simulink model "Work3"  (R2015b)
settings: Solver=FixedStepAuto  SolverMode=SingleTasking  StartTime=0.0  StopTime=20  FixedStep=0.01  RelTol=1e-3
values from neighbouring files (symbols this model uses):
  diff = 4    [diff.mat]
  diff2 = 240    [diff2.mat]
  Integ = 1.89    [Integ.mat]
  Integ2 = 1.6    [Integ2.mat]
  P = 8    [P.mat]
  P2 = 360    [P2.mat]
undefined symbols (not defined in the file or in its folder): ss1, ss2
settings Model: ExtModeTrigDuration=2  Creator=Druzhinin_Vasily  LastModifiedBy=Druzhinin_Vasily
settings OptimizationCC: DefaultParameterBehavior=Inlined  UseFloatMulNetSlope=on  InlineInvariantSignals=on  PassReuseOutputArgsAs=Individual arguments  ZeroExternalMemoryAtStartup=off  ZeroInternalMemoryAtStartup=off  NoFixptDivByZeroProtection=on  EfficientFloat2IntCast=on  OptimizeModelRefInitCode=on  LifeSpan=1  MaxStackSize=64
settings RTWCC: SystemTargetFile=ert.tlc  TemplateMakefile=ert_default_tmf  Description=Embedded Coder  GenerateReport=on  Toolchain=Arduino AVR v1.6.1  BuildConfiguration=Faster Runs  IncludeHyperlinkInReport=on  LaunchReport=on  GenerateTraceInfo=on  GenerateTraceReport=on  GenerateTraceReportSl=on  GenerateTraceReportSf=on  GenerateTraceReportEml=on  GenerateCodeMetricsReport=on
settings CodeAppCC: ForceParamTrailComments=on  IgnoreCustomStorageClasses=off  SimulinkDataObjDesc=on  CustomSymbolStrGlobalVar=rt$N$M  CustomSymbolStrType=$N$M  CustomSymbolStrFcn=$N$M$F  CustomSymbolStrMacro=$N$M  InsertBlockDesc=on
settings ERTTargetCC: IncludeMdlTerminateFcn=off  CombineSignalStateStructs=on  SupportContinuousTime=on  SupportVariableSizeSignals=on  InlinedParameterPlacement=NonHierarchical  ERTCustomFileTemplate=example_file_process.tlc  ERTFilePackagingFormat=CompactWithDataFile

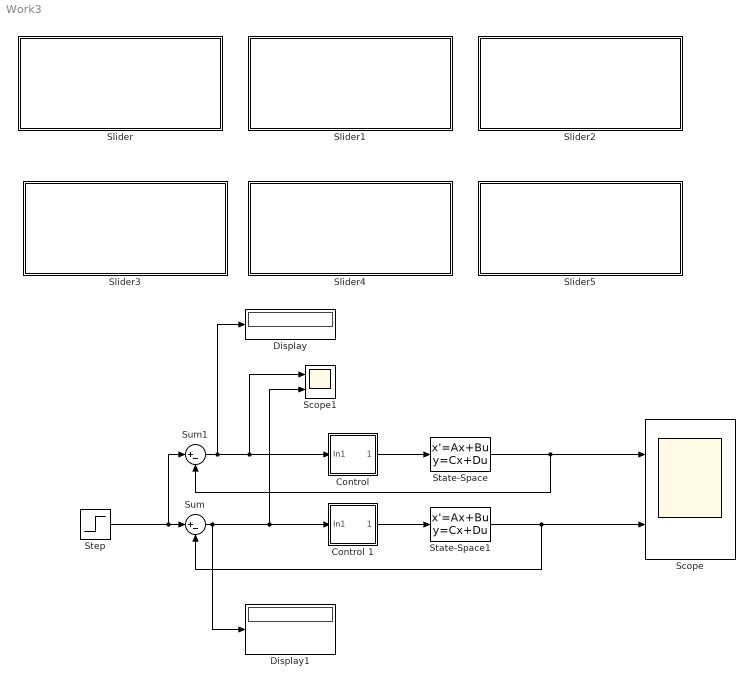
== system Work3 ==
  "Control " : Subsystem
  Control 1 : Subsystem
  Display : Display
  Display1 : Display
  Scope : Scope  NumInputPorts=2
  Scope1 : Scope  NumInputPorts=2
  Slider : Subsystem  DialogController=hmiCreateDDGDialog  IsWebBlock=on  mask(MWDashboardBlock){webBlockId=fcde2a52-5679-498e-b0b0-f5f8bdaff23e, webBlockType=slider, ShowInLibBrowser=on, ShowInitialText=on, HMISrcModelName=Work3}
      mask prompts: webBlockId "WebBlock Id"; webBlockType "WebBlock Type"; HMISrcModelName "Source Model"
      mask Help: helpview([docroot '/mapfiles/simulink.map'], 'hmi_slider')
      mask Display:
      | if strcmp(get_param(bdroot(gcb),'BlockDiagramType'), 'library')
      |     image([(matlabroot) '/toolbox/simulink/hmi/icons/Slider.png']);
      | end
  Slider1 : Subsystem  DialogController=hmiCreateDDGDialog  IsWebBlock=on  mask(MWDashboardBlock){webBlockId=34f26c4b-778d-474b-b420-5e3debdaa527, webBlockType=slider, ShowInLibBrowser=on, ShowInitialText=on, HMISrcModelName=Work3}
      mask prompts: webBlockId "WebBlock Id"; webBlockType "WebBlock Type"; HMISrcModelName "Source Model"
      mask Help: helpview([docroot '/mapfiles/simulink.map'], 'hmi_slider')
      mask Display:
      | if strcmp(get_param(bdroot(gcb),'BlockDiagramType'), 'library')
      |     image([(matlabroot) '/toolbox/simulink/hmi/icons/Slider.png']);
      | end
  Slider2 : Subsystem  DialogController=hmiCreateDDGDialog  IsWebBlock=on  mask(MWDashboardBlock){webBlockId=5f60686c-b0fe-4f18-a9e2-fcd4e663f137, webBlockType=slider, ShowInLibBrowser=on, ShowInitialText=on, HMISrcModelName=Work3}
      mask prompts: webBlockId "WebBlock Id"; webBlockType "WebBlock Type"; HMISrcModelName "Source Model"
      mask Help: helpview([docroot '/mapfiles/simulink.map'], 'hmi_slider')
      mask Display:
      | if strcmp(get_param(bdroot(gcb),'BlockDiagramType'), 'library')
      |     image([(matlabroot) '/toolbox/simulink/hmi/icons/Slider.png']);
      | end
  Slider3 : Subsystem  DialogController=hmiCreateDDGDialog  IsWebBlock=on  mask(MWDashboardBlock){webBlockId=a2bf55c6-834c-4e95-99ad-44c455448221, webBlockType=slider, ShowInLibBrowser=on, ShowInitialText=on, HMISrcModelName=Work3}
      mask prompts: webBlockId "WebBlock Id"; webBlockType "WebBlock Type"; HMISrcModelName "Source Model"
      mask Help: helpview([docroot '/mapfiles/simulink.map'], 'hmi_slider')
      mask Display:
      | if strcmp(get_param(bdroot(gcb),'BlockDiagramType'), 'library')
      |     image([(matlabroot) '/toolbox/simulink/hmi/icons/Slider.png']);
      | end
  Slider4 : Subsystem  DialogController=hmiCreateDDGDialog  IsWebBlock=on  mask(MWDashboardBlock){webBlockId=93ab61cf-ceae-4acd-b5ad-db12f044e680, webBlockType=slider, ShowInLibBrowser=on, ShowInitialText=on, HMISrcModelName=Work3}
      mask prompts: webBlockId "WebBlock Id"; webBlockType "WebBlock Type"; HMISrcModelName "Source Model"
      mask Help: helpview([docroot '/mapfiles/simulink.map'], 'hmi_slider')
      mask Display:
      | if strcmp(get_param(bdroot(gcb),'BlockDiagramType'), 'library')
      |     image([(matlabroot) '/toolbox/simulink/hmi/icons/Slider.png']);
      | end
  Slider5 : Subsystem  DialogController=hmiCreateDDGDialog  IsWebBlock=on  mask(MWDashboardBlock){webBlockId=0c8f17bd-0089-4b6b-8033-3296dc0310bd, webBlockType=slider, ShowInLibBrowser=on, ShowInitialText=on, HMISrcModelName=Work3}
      mask prompts: webBlockId "WebBlock Id"; webBlockType "WebBlock Type"; HMISrcModelName "Source Model"
      mask Help: helpview([docroot '/mapfiles/simulink.map'], 'hmi_slider')
      mask Display:
      | if strcmp(get_param(bdroot(gcb),'BlockDiagramType'), 'library')
      |     image([(matlabroot) '/toolbox/simulink/hmi/icons/Slider.png']);
      | end
  State-Space : StateSpace  A=ss1.A  B=ss1.B  C=ss1.C  D=ss1.D  X0=0
  State-Space1 : StateSpace  A=ss2.A  B=ss2.B  C=ss2.C  D=ss2.D  X0=0
  Step : Step  SampleTime=0
  Sum : Sum  Inputs=|+-
  Sum1 : Sum  Inputs=|+-
  wires:
  State-Space/1 -> Sum1/2, Scope/1
  Step/1 -> Sum/1, Sum1/1
  State-Space1/1 -> Sum/2, Scope/2
  Sum/1 -> Display1/1, Control 1/1(In1), Scope1/2
  Sum1/1 -> Display/1, "Control "/1(In1), Scope1/1
  Control 1/1(Out1) -> State-Space1/1
  "Control "/1(Out1) -> State-Space/1

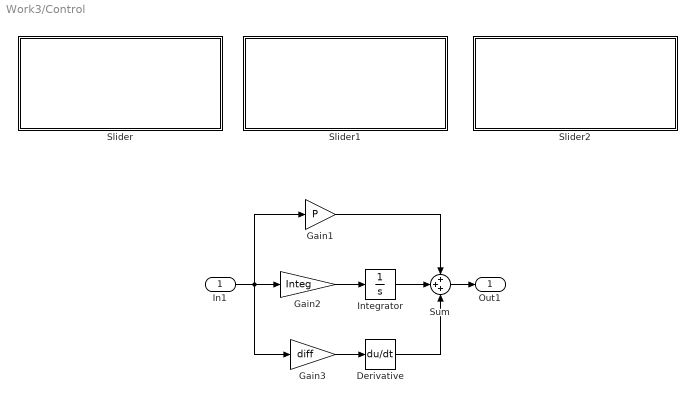
== system Work3/Control  ==
  In1 : Inport
  Derivative : Derivative
  Gain1 : Gain  Gain=P
  Gain2 : Gain  Gain=Integ
  Gain3 : Gain  Gain=diff
  Integrator : Integrator
  Slider : Subsystem  DialogController=hmiCreateDDGDialog  IsWebBlock=on  mask(MWDashboardBlock){webBlockId=3970b7c4-10f1-407d-9023-fc3db7863d85, webBlockType=slider, ShowInLibBrowser=on, ShowInitialText=on, HMISrcModelName=Work3}
      mask prompts: webBlockId "WebBlock Id"; webBlockType "WebBlock Type"; HMISrcModelName "Source Model"
      mask Help: helpview([docroot '/mapfiles/simulink.map'], 'hmi_slider')
      mask Display:
      | if strcmp(get_param(bdroot(gcb),'BlockDiagramType'), 'library')
      |     image([(matlabroot) '/toolbox/simulink/hmi/icons/Slider.png']);
      | end
  Slider1 : Subsystem  DialogController=hmiCreateDDGDialog  IsWebBlock=on  mask(MWDashboardBlock){webBlockId=385fd4e2-0816-4699-9fa8-c3dc2c8cdf68, webBlockType=slider, ShowInLibBrowser=on, ShowInitialText=on, HMISrcModelName=Work3}
      mask prompts: webBlockId "WebBlock Id"; webBlockType "WebBlock Type"; HMISrcModelName "Source Model"
      mask Help: helpview([docroot '/mapfiles/simulink.map'], 'hmi_slider')
      mask Display:
      | if strcmp(get_param(bdroot(gcb),'BlockDiagramType'), 'library')
      |     image([(matlabroot) '/toolbox/simulink/hmi/icons/Slider.png']);
      | end
  Slider2 : Subsystem  DialogController=hmiCreateDDGDialog  IsWebBlock=on  mask(MWDashboardBlock){webBlockId=c188513b-0204-41a7-abc6-dab192722c83, webBlockType=slider, ShowInLibBrowser=on, ShowInitialText=on, HMISrcModelName=Work3}
      mask prompts: webBlockId "WebBlock Id"; webBlockType "WebBlock Type"; HMISrcModelName "Source Model"
      mask Help: helpview([docroot '/mapfiles/simulink.map'], 'hmi_slider')
      mask Display:
      | if strcmp(get_param(bdroot(gcb),'BlockDiagramType'), 'library')
      |     image([(matlabroot) '/toolbox/simulink/hmi/icons/Slider.png']);
      | end
  Sum : Sum  Inputs=+++
  Out1 : Outport
  wires:
  Sum/1 -> Out1/1
  Gain2/1 -> Integrator/1
  Gain3/1 -> Derivative/1
  Gain1/1 -> Sum/1
  In1/1 -> Gain1/1, Gain3/1, Gain2/1
  Integrator/1 -> Sum/2
  Derivative/1 -> Sum/3

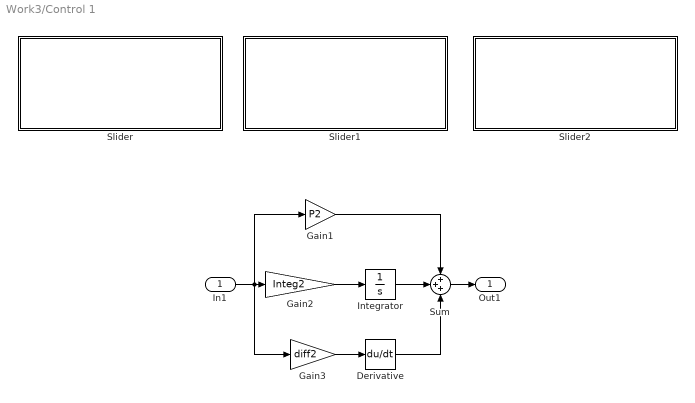
== system Work3/Control 1 ==
  In1 : Inport
  Derivative : Derivative
  Gain1 : Gain  Gain=P2
  Gain2 : Gain  Gain=Integ2
  Gain3 : Gain  Gain=diff2
  Integrator : Integrator
  Slider : Subsystem  DialogController=hmiCreateDDGDialog  IsWebBlock=on  mask(MWDashboardBlock){webBlockId=676329b8-bdc0-4adf-8661-756c4859d241, webBlockType=slider, ShowInLibBrowser=on, ShowInitialText=on, HMISrcModelName=Work3}
      mask prompts: webBlockId "WebBlock Id"; webBlockType "WebBlock Type"; HMISrcModelName "Source Model"
      mask Help: helpview([docroot '/mapfiles/simulink.map'], 'hmi_slider')
      mask Display:
      | if strcmp(get_param(bdroot(gcb),'BlockDiagramType'), 'library')
      |     image([(matlabroot) '/toolbox/simulink/hmi/icons/Slider.png']);
      | end
  Slider1 : Subsystem  DialogController=hmiCreateDDGDialog  IsWebBlock=on  mask(MWDashboardBlock){webBlockId=570aac75-bd02-46f0-a613-92906a6ffe1d, webBlockType=slider, ShowInLibBrowser=on, ShowInitialText=on, HMISrcModelName=Work3}
      mask prompts: webBlockId "WebBlock Id"; webBlockType "WebBlock Type"; HMISrcModelName "Source Model"
      mask Help: helpview([docroot '/mapfiles/simulink.map'], 'hmi_slider')
      mask Display:
      | if strcmp(get_param(bdroot(gcb),'BlockDiagramType'), 'library')
      |     image([(matlabroot) '/toolbox/simulink/hmi/icons/Slider.png']);
      | end
  Slider2 : Subsystem  DialogController=hmiCreateDDGDialog  IsWebBlock=on  mask(MWDashboardBlock){webBlockId=20f6314d-6e10-4601-8f41-e12dac693f5f, webBlockType=slider, ShowInLibBrowser=on, ShowInitialText=on, HMISrcModelName=Work3}
      mask prompts: webBlockId "WebBlock Id"; webBlockType "WebBlock Type"; HMISrcModelName "Source Model"
      mask Help: helpview([docroot '/mapfiles/simulink.map'], 'hmi_slider')
      mask Display:
      | if strcmp(get_param(bdroot(gcb),'BlockDiagramType'), 'library')
      |     image([(matlabroot) '/toolbox/simulink/hmi/icons/Slider.png']);
      | end
  Sum : Sum  Inputs=+++
  Out1 : Outport
  wires:
  Derivative/1 -> Sum/3
  Integrator/1 -> Sum/2
  In1/1 -> Gain2/1, Gain3/1, Gain1/1
  Gain1/1 -> Sum/1
  Gain3/1 -> Derivative/1
  Gain2/1 -> Integrator/1
  Sum/1 -> Out1/1

== system Work3/Slider ==

== system Work3/Slider1 ==

== system Work3/Slider2 ==

== system Work3/Slider3 ==

== system Work3/Slider4 ==

== system Work3/Slider5 ==

== system Work3/Control /Slider ==

== system Work3/Control /Slider1 ==

== system Work3/Control /Slider2 ==

== system Work3/Control 1/Slider ==

== system Work3/Control 1/Slider1 ==

== system Work3/Control 1/Slider2 ==
